simulink model "TestLevel_2_MODEL"  (R2017b)
settings: Solver=VariableStepAuto  StartTime=0.0  StopTime=20000000  MaxStep=200  RelTol=1e-3
libraries: instrumentlib x2, svdutilitieslib x1
settings Model: Creator=Bruger  LastModifiedBy=koch

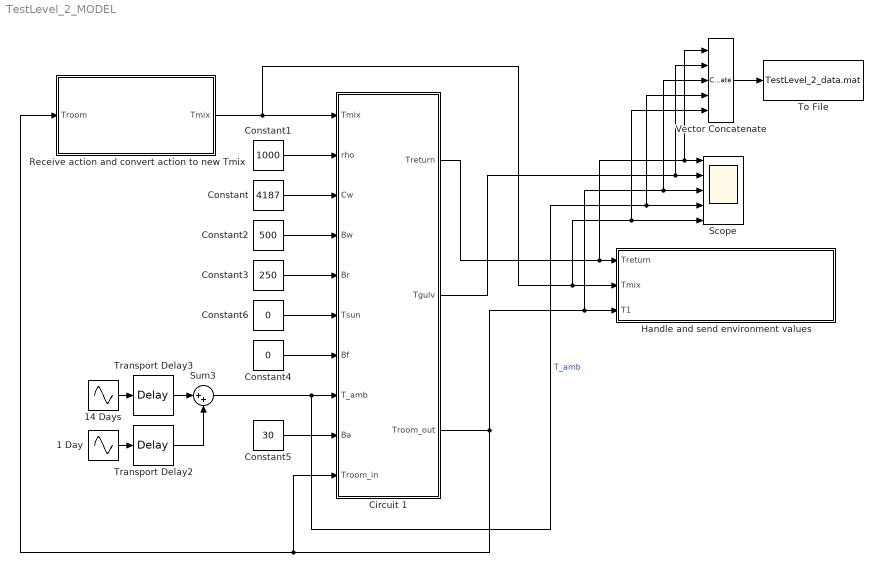
== system TestLevel_2_MODEL ==
  1 Day : Sin  Amplitude=4  Frequency=0.00007272205216643  SampleTime=0
  14 Days : Sin  Amplitude=2  Frequency=0.00000519443  SampleTime=0
  Circuit 1 : Subsystem
  Constant : Constant  Value=4187
  Constant1 : Constant  Value=1000
  Constant2 : Constant  Value=500
  Constant3 : Constant  Value=250
  Constant4 : Constant  Value=0
  Constant5 : Constant  Value=30
  Constant6 : Constant  Value=0
  Handle and send environment values : Subsystem
  Receive action and convert action to new Tmix : Subsystem
  Scope : Scope  NumInputPorts=5
  Sum3 : Sum  Inputs=|++
  To File : ToFile  Filename=TestLevel_2_data.mat  SaveFormat=Timeseries
  Transport Delay2 : TransportDelay  DelayTime=15000000
  Transport Delay3 : TransportDelay  DelayTime=10000000
  Vector Concatenate : Concatenate  NumInputs=5
  wires:
  14 Days/1 -> Transport Delay3/1
  Sum3/1 -> Vector Concatenate/4, Scope/4, Circuit 1/8(T_amb)  "T_amb"
  1 Day/1 -> Transport Delay2/1
  Transport Delay3/1 -> Sum3/1
  Transport Delay2/1 -> Sum3/2
  Vector Concatenate/1 -> To File/1
  Receive action and convert action to new Tmix/1(Tmix) -> Circuit 1/1(Tmix), Vector Concatenate/5, Scope/5, Handle and send environment values/2(Tmix)
  Circuit 1/1(Treturn) -> Vector Concatenate/1, Scope/1, Handle and send environment values/1(Treturn)
  Circuit 1/3(Troom_out) -> Receive action and convert action to new Tmix/1(Troom), Circuit 1/10(Troom_in), Vector Concatenate/3, Scope/3, Handle and send environment values/3(T1)
  Constant1/1 -> Circuit 1/2(rho)
  Constant/1 -> Circuit 1/3(Cw)
  Constant2/1 -> Circuit 1/4(Bw)
  Constant3/1 -> Circuit 1/5(Br)
  Constant6/1 -> Circuit 1/6(Tsun)
  Constant4/1 -> Circuit 1/7(Bf)
  Constant5/1 -> Circuit 1/9(Ba)
  Circuit 1/2(Tgulv) -> Vector Concatenate/2, Scope/2

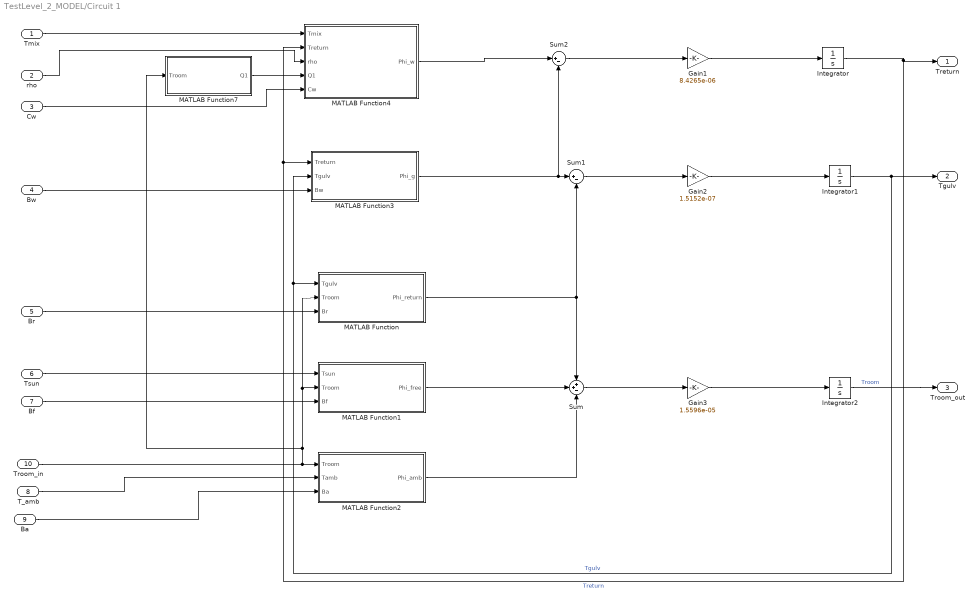
== system TestLevel_2_MODEL/Circuit 1 ==
  Tmix : Inport
  rho : Inport  Port=2
  Cw : Inport  Port=3
  Bw : Inport  Port=4
  Br : Inport  Port=5
  Tsun : Inport  Port=6
  Bf : Inport  Port=7
  T_amb : Inport  Port=8
  Ba : Inport  Port=9
  Troom_in : Inport  Port=10
  Gain1 : Gain  Gain=8.4265e-06
  Gain2 : Gain  Gain=1.5152e-07
  Gain3 : Gain  Gain=1.5596e-05
  Integrator : Integrator  InitialCondition=16
  Integrator1 : Integrator  InitialCondition=16
  Integrator2 : Integrator  InitialCondition=16
  MATLAB Function : MATLAB Function  TreatAsAtomicUnit=on
  MATLAB Function1 : MATLAB Function  TreatAsAtomicUnit=on
  MATLAB Function2 : MATLAB Function  TreatAsAtomicUnit=on
  MATLAB Function3 : MATLAB Function  TreatAsAtomicUnit=on
  MATLAB Function4 : MATLAB Function  TreatAsAtomicUnit=on
  MATLAB Function7 : MATLAB Function  TreatAsAtomicUnit=on
  Sum : Sum  Inputs=++-
  Sum1 : Sum  Inputs=|+-
  Sum2 : Sum  Inputs=|+-
  Treturn : Outport
  Tgulv : Outport  Port=2
  Troom_out : Outport  Port=3
  wires:
  MATLAB Function1/1(Phi_free) -> Sum/2
  MATLAB Function4/1(Phi_w) -> Sum2/1
  MATLAB Function7/1(Q1) -> MATLAB Function4/4(Q1)
  MATLAB Function2/1(Phi_amb) -> Sum/3
  Sum2/1 -> Gain1/1
  Bf/1 -> MATLAB Function1/3(Bf)
  Integrator1/1 -> MATLAB Function/1(Tgulv), MATLAB Function3/2(Tgulv), Tgulv/1  "Tgulv"
  Integrator2/1 -> Troom_out/1  "Troom"
  MATLAB Function3/1(Phi_g) -> Sum2/2, Sum1/1
  MATLAB Function/1(Phi_return) -> Sum/1, Sum1/2
  Bw/1 -> MATLAB Function3/3(Bw)
  Cw/1 -> MATLAB Function4/5(Cw)
  rho/1 -> MATLAB Function4/3(rho)
  Sum1/1 -> Gain2/1
  Gain1/1 -> Integrator/1
  Gain2/1 -> Integrator1/1
  Integrator/1 -> MATLAB Function4/2(Treturn), MATLAB Function3/1(Treturn), Treturn/1  "Treturn"
  Tsun/1 -> MATLAB Function1/1(Tsun)
  Gain3/1 -> Integrator2/1
  Ba/1 -> MATLAB Function2/3(Ba)
  Br/1 -> MATLAB Function/3(Br)
  Sum/1 -> Gain3/1
  Troom_in/1 -> MATLAB Function2/1(Troom), MATLAB Function7/1(Troom), MATLAB Function/2(Troom), MATLAB Function1/2(Troom)
  Tmix/1 -> MATLAB Function4/1(Tmix)
  T_amb/1 -> MATLAB Function2/2(Tamb)

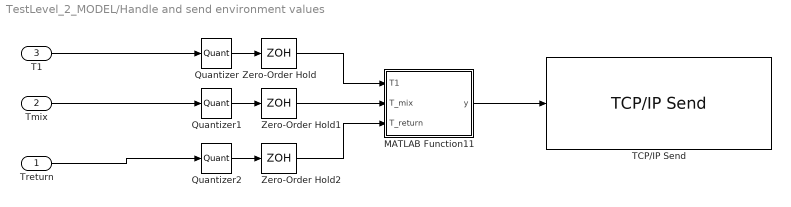
== system TestLevel_2_MODEL/Handle and send environment values ==
  Treturn : Inport
  Tmix : Inport  Port=2
  T1 : Inport  Port=3
  MATLAB Function11 : MATLAB Function  TreatAsAtomicUnit=on
  Quantizer : Quantizer  QuantizationInterval=0.01
  Quantizer1 : Quantizer  QuantizationInterval=0.01
  Quantizer2 : Quantizer  QuantizationInterval=0.01
  TCP/IP Send : instrumentlib/TCP//IP Send  Priority=2  Host=localhost  Port=50001  EnableBlockingMode=on  Timeout=10  ByteOrder=LittleEndian
      settings: SourceProductName=Instrument Control Toolbox
  Zero-Order Hold : ZeroOrderHold  SampleTime=-1
  Zero-Order Hold1 : ZeroOrderHold  SampleTime=-1
  Zero-Order Hold2 : ZeroOrderHold  SampleTime=-1
  wires:
  Quantizer1/1 -> Zero-Order Hold1/1
  Quantizer/1 -> Zero-Order Hold/1
  Quantizer2/1 -> Zero-Order Hold2/1
  Zero-Order Hold1/1 -> MATLAB Function11/2(T_mix)
  Zero-Order Hold/1 -> MATLAB Function11/1(T1)
  Zero-Order Hold2/1 -> MATLAB Function11/3(T_return)
  MATLAB Function11/1(y) -> TCP/IP Send/1
  Tmix/1 -> Quantizer1/1
  T1/1 -> Quantizer/1
  Treturn/1 -> Quantizer2/1

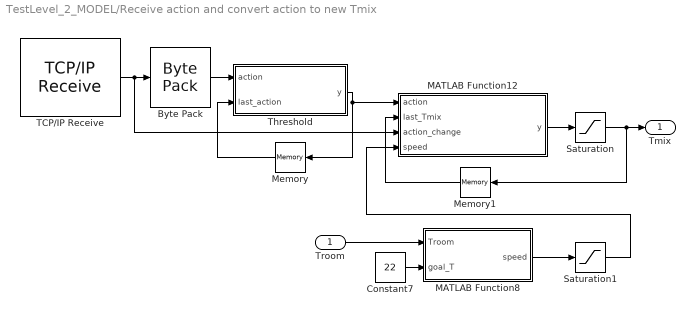
== system TestLevel_2_MODEL/Receive action and convert action to new Tmix ==
  Troom : Inport
  Byte Pack : svdutilitieslib/Byte Pack  datatypes={'uint8'}  byteAlign=1  blockPlatform=arduinoert
      settings: SourceProductName=Simulink Support Package for Arduino Hardware  SourceProductBaseCode=ARDUINO
  Constant7 : Constant  Value=22
  MATLAB Function12 : MATLAB Function  TreatAsAtomicUnit=on
  MATLAB Function8 : MATLAB Function  TreatAsAtomicUnit=on
  Memory : Memory
  Memory1 : Memory  InitialCondition=24
  Saturation : Saturate  UpperLimit=45  LowerLimit=15
  Saturation1 : Saturate  UpperLimit=0.8  LowerLimit=0.005
  TCP/IP Receive : instrumentlib/TCP//IP Receive  Host=localhost  Port=50000  DataSize=[1 1]  EnableBlockingMode=on  Timeout=15  SampleTime=200  DataType=uint8  ByteOrder=BigEndian
      settings: SourceProductName=Instrument Control Toolbox
  Threshold : MATLAB Function  TreatAsAtomicUnit=on
  Tmix : Outport
  wires:
  MATLAB Function12/1(y) -> Saturation/1
  TCP/IP Receive/1 -> MATLAB Function12/3(action_change), Byte Pack/1
  Threshold/1(y) -> MATLAB Function12/1(action), Memory/1
  MATLAB Function8/1(speed) -> Saturation1/1
  Saturation1/1 -> MATLAB Function12/4(speed)
  Memory/1 -> Threshold/2(last_action)
  Saturation/1 -> Tmix/1, Memory1/1
  Byte Pack/1 -> Threshold/1(action)
  Constant7/1 -> MATLAB Function8/2(goal_T)
  Memory1/1 -> MATLAB Function12/2(last_Tmix)
  Troom/1 -> MATLAB Function8/1(Troom)

== matlab function TestLevel_2_MODEL/Circuit 1/MATLAB Function1 ==
  data: Tsun input; Phi_free output; Troom input; Bf input
function Phi_free = fcn(Tsun,Troom,Bf)

Phi_free = Bf * ( Tsun-Troom)

== matlab function TestLevel_2_MODEL/Circuit 1/MATLAB Function ==
  data: Tgulv input; Phi_return output; Troom input; Br input
function Phi_return = fcn(Tgulv,Troom,Br)

Phi_return = Br * ( Tgulv-Troom)

== matlab function TestLevel_2_MODEL/Circuit 1/MATLAB Function2 ==
  data: Troom input; Tamb input; Phi_amb output; Ba input
function Phi_amb = fcn(Troom,Tamb,Ba)

Phi_amb = Ba * ( Troom-Tamb)

== matlab function TestLevel_2_MODEL/Circuit 1/MATLAB Function3 ==
  data: Treturn input; Tgulv input; Phi_g output; Bw input
function Phi_g= fcn(Treturn,Tgulv,Bw)

Phi_g = Bw * ( Treturn-Tgulv)

== matlab function TestLevel_2_MODEL/Circuit 1/MATLAB Function4 ==
  data: Tmix input; Treturn input; Phi_w output; rho input; Q1 input; Cw input
function Phi_w= fcn(Tmix,Treturn,rho,Q1,Cw)

Phi_w = rho*Q1 *Cw* ( Tmix-Treturn)

== matlab function TestLevel_2_MODEL/Circuit 1/MATLAB Function7 ==
  data: Troom input; Q1 output
function Q1 = fcn(Troom)

if Troom < 20
    Q1 = 0.000027777778
else 
    Q1 = 0.000027777778 
end

== matlab function TestLevel_2_MODEL/Receive action and convert action to new Tmix/MATLAB Function8 ==
  data: speed output; Troom input; goal_T input
function speed = fcn(Troom, goal_T)

if goal_T > 0 && Troom > 0
    speed = abs(goal_T - Troom)*1.5;
else 
    speed = 0.1;
end

if speed < 0.03
    speed =0.03;
end

== matlab function TestLevel_2_MODEL/Handle and send environment values/MATLAB Function11 ==
  data: T1 input; y output; T_mix input; T_return input
function y = fcn(T1, T_mix, T_return)


y = [T1,4.5,4.6,4.7,T_mix,T_return];

== matlab function TestLevel_2_MODEL/Receive action and convert action to new Tmix/MATLAB Function12 ==
  data: action input; y output; last_Tmix input; action_change input; speed input
function y = fcn(action, last_Tmix, action_change, speed)

%Only make change if a action is received by the TCP/IP receiver
if action_change > 0 
    k = 1;
else
    k = 0;
end


if action < 2 && k>0
    y = last_Tmix;
    k = 0;
elseif 1 < action && action < 3 && k>0
    y = last_Tmix - speed;
    k = 0;
elseif 2 < action && k>0
    y = last_Tmix+speed;
    k = 0;
elseif action > 20
    y = action;
else
    y = last_Tmix;
end

== matlab function TestLevel_2_MODEL/Receive action and convert action to new Tmix/Threshold ==
  data: action input; y output; last_action input
function y  = fcn(action,last_action)

action = double(action);
% zero is not a option so
if action > 0
    y = action;
else
    y = last_action;
end
